simulink model "Braking_System_2021b"  (R2021b)
settings: Solver=VariableStepAuto  StartTime=0.0  StopTime=10.0  RelTol=1e-3
undefined symbols (not defined in the file): booster_calcData, booster_k1, booster_k2, Fp, frontBrake_cfrbr, lagtime, maitre_cyl_calcData, MR_trgtDecc_Unbrked, MR_trgtMass_Unbrked, Pa_max_ax, Pa_max_b, Pa_min_ax, Pa_min_b, pedale_calcData, pedale_Fr, pedale_method, pedale_Ratio_Test, pedale_Rp, pedale_TEST, Tf_ax, Tf_b, tracteur_chargeAR, tracteur_chargeAV, tracteur_h, tracteur_masseLaden, tracteur_masseLadenAR, tracteur_masseLadenAV, tracteur_masseUnladen, tracteur_masseUnladenAR, tracteur_masseUnladenAV, tracteur_maxRayAR, tracteur_maxRayAV, tracteur_minRayAR, tracteur_minRayAV, tracteur_RollRes, tracteur_x1, tracteur_x2, transmission_calcData, transmission_R4wd, transmission_Rbs, transmission_Redn_AV, transmission_Rend_AR, transmission_Rend_AV, transmission_Rfa, transmission_Rra, valve_hp_calcData, valve_hp_k1, valve_hp_k2, vitesse
libraries: simulink x2
settings Model: Creator=sb74808  LastModifiedBy=sb74808
settings DebuggingCC: UnconnectedInputMsg=none  UnconnectedOutputMsg=none  UnconnectedLineMsg=none
settings ModelReferenceCC: EnableRefExpFcnMdlSchedulingChecks=off
settings RTWCC: DLArmComputeVersion=20.02.1

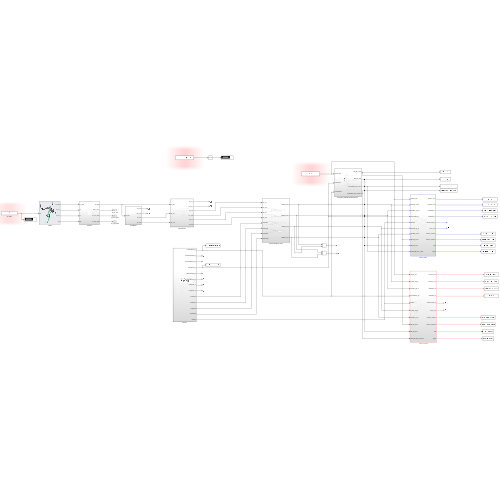
[thumbnail: Simulink's stored preview of the top-level diagram]
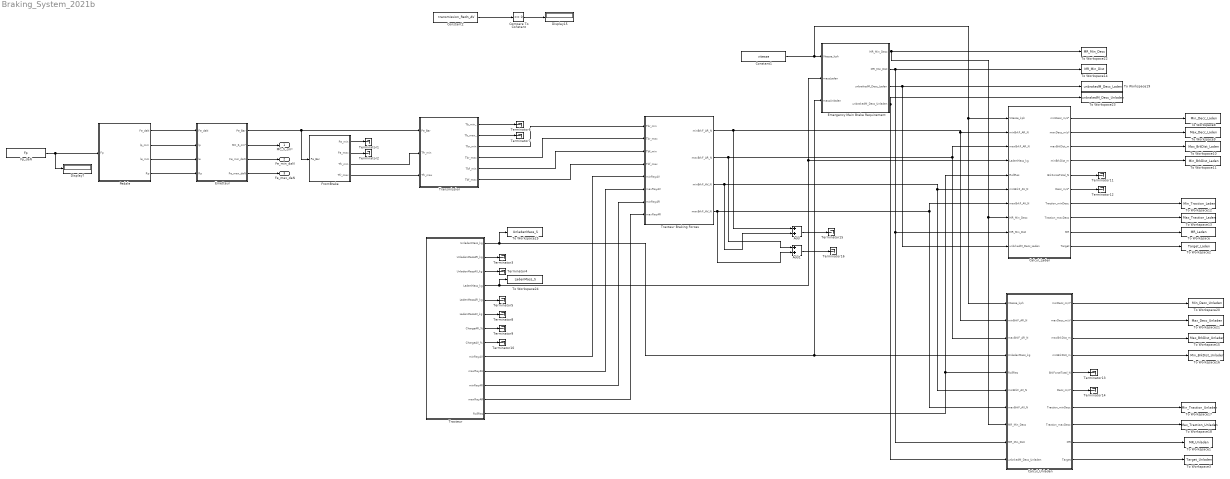
== system Braking_System_2021b ==
  Add : Sum
  Add1 : Sum
  Calcul_Laden : Subsystem
  Calcul_Unladen : Subsystem
  Compare To Constant : simulink/Logic and Bit Operations/Compare To Constant  relop===  const=0  OutDataTypeStr=boolean
  Constant1 : Constant  Value=vitesse
  Constant2 : Constant  Value=transmission_Redn_AV
  Display15 : Display
  Display7 : Display
  Emergency Main Brake Requirement : Subsystem
  Emetteur : Subsystem
  Fp_daN : Constant  Value=Fp
  FrontBrake : Subsystem
  Pedale : Subsystem
      mask Display: image('C:\Users\sb74808\OneDrive - AGCO Corp\Bureau\pedal.png'); % Use "Edit Image" on toolstrip to change.
  Terminator{1..16} (16 alike) : Terminator
  To Workspace : ToWorkspace  VariableName=MR_Laden  SaveFormat=Structure  SampleTime=-1
  To Workspace1 : ToWorkspace  VariableName=MR_Unladen  SaveFormat=Structure  SampleTime=-1
  To Workspace10 : ToWorkspace  VariableName=Max_BrkDist_Laden  SaveFormat=Structure  SampleTime=-1
  To Workspace11 : ToWorkspace  VariableName=Min_BrkDist_Laden  SaveFormat=Structure  SampleTime=-1
  To Workspace12 : ToWorkspace  VariableName=Min_Traction_Laden  SaveFormat=Structure  SampleTime=-1
      settings: Save2DSignal=2-D array (concatenate along first dimension)
  To Workspace13 : ToWorkspace  VariableName=Max_Traction_Laden  SaveFormat=Structure  SampleTime=-1
  To Workspace14 : ToWorkspace  VariableName=MR_Min_Dist  SaveFormat=Structure  SampleTime=-1
  To Workspace15 : ToWorkspace  VariableName=Max_BrkDist_Unladen  SaveFormat=Structure  SampleTime=-1
  To Workspace16 : ToWorkspace  VariableName=Min_BrkDist_Unladen  SaveFormat=Structure  SampleTime=-1
  To Workspace17 : ToWorkspace  VariableName=Min_Traction_Unladen  SaveFormat=Structure  SampleTime=-1
  To Workspace18 : ToWorkspace  VariableName=Max_Traction_Unladen  SaveFormat=Structure  SampleTime=-1
  To Workspace19 : ToWorkspace  VariableName=unbrakedM_Decc_Laden  SaveFormat=Structure  SampleTime=-1
  To Workspace2 : ToWorkspace  VariableName=Target_Laden  SaveFormat=Structure  SampleTime=-1
  To Workspace20 : ToWorkspace  VariableName=Min_Decc_Unladen  SaveFormat=Structure  SampleTime=-1
  To Workspace21 : ToWorkspace  VariableName=Max_Decc_Unladen  SaveFormat=Structure  SampleTime=-1
  To Workspace22 : ToWorkspace  VariableName=MR_Min_Decc  SaveFormat=Structure  SampleTime=-1
  To Workspace23 : ToWorkspace  VariableName=unbrakedM_Decc_Unladen  SaveFormat=Structure  SampleTime=-1
  To Workspace24 : ToWorkspace  VariableName=LadenMass_S  SaveFormat=Structure  SampleTime=-1
  To Workspace25 : ToWorkspace  VariableName=UnladenMass_S  SaveFormat=Structure  SampleTime=-1
  To Workspace3 : ToWorkspace  VariableName=Target_Unladen  SaveFormat=Structure  SampleTime=-1
  To Workspace8 : ToWorkspace  VariableName=Min_Decc_Laden  SaveFormat=Structure  SampleTime=-1
  To Workspace9 : ToWorkspace  VariableName=Max_Decc_Laden  SaveFormat=Structure  SampleTime=-1
  Tracteur : Subsystem
  Tracteur Braking Forces : Subsystem
  Transmission : Subsystem
  MC_S_cm² : Outport
  Fe_min_daN : Outport  Port=2
  Fe_max_daN : Outport  Port=3
  wires:
  Fp_daN/1 -> Pedale/1(Fp), Display7/1
  Pedale/2(lp_mm) -> Emetteur/2(lp)
  Pedale/3(le_mm) -> Emetteur/3(le)
  Pedale/4(Rp) -> Emetteur/4(Rp)
  Pedale/1(Fe_daN) -> Emetteur/1(Fe_daN)
  Emetteur/2(MC_S_cm²) -> MC_S_cm²/1
  Emetteur/3(Fe_min_daN) -> Fe_min_daN/1
  Emetteur/4(Fe_max_daN) -> Fe_max_daN/1
  Emetteur/1(Pe_Bar) -> FrontBrake/1(Pe_Bar), Transmission/1(Pe_Bar)
  FrontBrake/4(Tfr_max) -> Transmission/3(Tfr_max)
  FrontBrake/3(Tfr_min) -> Transmission/2(Tfr_min)
  Compare To Constant/1 -> Display15/1
  Constant2/1 -> Compare To Constant/1
  Transmission/3(Tbr_min) -> Tracteur Braking Forces/1(Tbr_min)
  Transmission/5(Tbf_min) -> Tracteur Braking Forces/3(Tbf_min)
  Transmission/6(Tbf_max) -> Tracteur Braking Forces/4(Tbf_max)
  Tracteur/9(minRayAV) -> Tracteur Braking Forces/5(minRayAV)
  Tracteur/10(maxRayAV) -> Tracteur Braking Forces/6(maxRayAV)
  Tracteur/11(minRayAR) -> Tracteur Braking Forces/7(minRayAR)
  Tracteur/12(maxRayAR) -> Tracteur Braking Forces/8(maxRayAR)
  Tracteur/13(RollRes) -> Calcul_Laden/5(RollRes), Calcul_Unladen/5(RollRes)
  Tracteur Braking Forces/1(minBrkF_AR_N) -> Add/1, Calcul_Unladen/2(minBrkF_AR_N), Calcul_Laden/2(minBrkF_AR_N)
  Tracteur Braking Forces/2(maxBrkF_AR_N) -> Calcul_Unladen/3(maxBrkF_AR_N), Calcul_Laden/3(maxBrkF_AR_N), Add1/1
  Tracteur Braking Forces/3(minBrkF_AV_N) -> Add/2, Calcul_Unladen/6(minBrkF_AV_N), Calcul_Laden/6(minBrkF_AV_N)
  Tracteur Braking Forces/4(maxBrkF_AV_N) -> Add1/2, Calcul_Unladen/7(maxBrkF_AV_N), Calcul_Laden/7(maxBrkF_AV_N)
  Transmission/1(Tb_min_) -> Terminator6/1
  Transmission/2(Tb_max_) -> Terminator7/1
  Transmission/4(Tbr_max) -> Tracteur Braking Forces/2(Tbr_max)
  Add/1 -> Terminator15/1
  Add1/1 -> Terminator16/1
  Constant1/1 -> Calcul_Unladen/1(Vitesse_kph), Calcul_Laden/1(Vitesse_kph), Emergency Main Brake Requirement/1(Vitesse_kph)
  Emergency Main Brake Requirement/1(MR_Min_Decc) -> To Workspace22/1, Calcul_Unladen/8(MR_Min_Decc), Calcul_Laden/8(MR_Min_Decc)
  Emergency Main Brake Requirement/2(MR_Min_Dist) -> To Workspace14/1, Calcul_Unladen/9(MR_Min_Dist), Calcul_Laden/9(MR_Min_Dist)
  Emergency Main Brake Requirement/3(unbrakedM_Decc_Laden) -> To Workspace19/1, Calcul_Laden/10(unbrkedM_Decc_Laden)
  Emergency Main Brake Requirement/4(unbrakedM_Decc_Unladen) -> To Workspace23/1, Calcul_Unladen/10(unbrkedM_Decc_Unladen)
  Calcul_Laden/1(minDecc_m/s²) -> To Workspace8/1
  Calcul_Laden/2(maxDecc_m/s²) -> To Workspace9/1
  Calcul_Laden/3(maxBrkDist_m) -> To Workspace10/1
  Calcul_Laden/4(minBrkDist_m) -> To Workspace11/1
  Calcul_Unladen/4(minBrkDist_m) -> To Workspace16/1
  Calcul_Unladen/3(maxBrkDist_m) -> To Workspace15/1
  Calcul_Unladen/2(maxDecc_m/s²) -> To Workspace21/1
  Calcul_Unladen/1(minDecc_m/s²) -> To Workspace20/1
  Tracteur/4(LadenMass_kg) -> Calcul_Laden/4(LadenMass_kg), Emergency Main Brake Requirement/2(massLaden), To Workspace24/1
  Tracteur/1(UnladenMass_kg) -> Calcul_Unladen/4(UnladenMass_kg), Emergency Main Brake Requirement/3(massUnladen), To Workspace25/1
  FrontBrake/1(Pa_min) -> Terminator1/1
  FrontBrake/2(Pa_max) -> Terminator2/1
  Tracteur/2(UnladenMassAR_kg) -> Terminator3/1
  Tracteur/3(UnladenMassAV_kg) -> Terminator4/1
  Tracteur/5(LadenMassAR_kg) -> Terminator5/1
  Tracteur/6(LadenMassAV_kg) -> Terminator8/1
  Tracteur/7(ChargeAR_%) -> Terminator9/1
  Tracteur/8(ChargeAV_%) -> Terminator10/1
  Calcul_Laden/5(BrkForceTotal_N) -> Terminator11/1
  Calcul_Laden/6(Decc_m/s²) -> Terminator12/1
  Calcul_Unladen/5(BrkForceTotal_N) -> Terminator13/1
  Calcul_Unladen/6(Decc_m/s²) -> Terminator14/1
  Calcul_Laden/9(MR) -> To Workspace/1
  Calcul_Laden/10(Target) -> To Workspace2/1
  Calcul_Laden/8(Traction_maxDecc) -> To Workspace13/1
  Calcul_Unladen/7(Traction_minDecc) -> To Workspace17/1
  Calcul_Unladen/8(Traction_maxDecc) -> To Workspace18/1
  Calcul_Unladen/9(MR) -> To Workspace1/1
  Calcul_Unladen/10(Target) -> To Workspace3/1
  Calcul_Laden/7(Traction_minDecc) -> To Workspace12/1

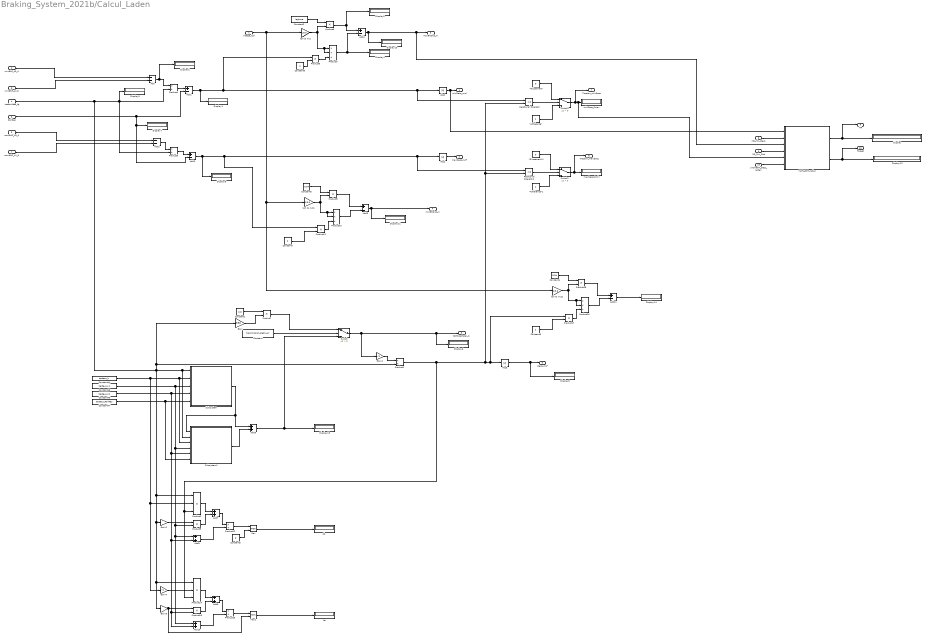
== system Braking_System_2021b/Calcul_Laden ==
  Vitesse_kph : Inport
  minBrkF_AR_N : Inport  Port=2
  maxBrkF_AR_N : Inport  Port=3
  LadenMass_kg : Inport  Port=4
  RollRes : Inport  Port=5
  minBrkF_AV_N : Inport  Port=6
  maxBrkF_AV_N : Inport  Port=7
  MR_Min_Decc : Inport  Port=8
  MR_Min_Dist : Inport  Port=9
  unbrkedM_Decc_Laden : Inport  Port=10
  "\"Adhérence\"" : Constant
  "\"Adhérence\"1" : Constant
  "\"Glissement\"" : Constant  Value=0
  "\"Glissement\"1" : Constant  Value=0
  Abs1 : Abs
  Abs2 : Abs
  Abs3 : Abs
  Add : Sum  Inputs=--
  Add{1,3..5,11} (5 alike) : Sum  Inputs=+-
  Add{6..10} (5 alike) : Sum
  Add2 : Sum  Inputs=--
  Constant : Constant  Value=transmission_Redn_AV
  Constant1 : Constant  Value=0.8
  Constant2 : Constant  Value=lagtime
  Constant3 : Constant  Value=0
  Constant4 : Constant  Value=0.54
  Constant44 : Constant  Value=tracteur_h
  Constant45 : Constant  Value=tracteur_x2
  Constant46 : Constant  Value=tracteur_x1
  Constant47 : Constant  Value=tracteur_RollRes
  Constant5 : Constant  Value=2
  Constant6 : Constant  Value=0.54
  Constant7 : Constant  Value=2
  Constant8 : Constant  Value=2
  Display{,1..14} (15 alike) : Display
  Gain : Gain  Gain=9.81
  Gain1 : Gain  Gain=-1
  Gain2 : Gain  Gain=9.81
  Gain3 : Gain  Gain=9.81
  Gain4 : Gain  Gain=-1
  MATLAB Function : MATLAB Function  TreatAsAtomicUnit=on
  Max : MinMax  Function=max  Inputs=2
  Max1 : MinMax  Inputs=2
  Na : Display
  Nb : Display
  Product{,3,6,8..9,11,15,17..18} (9 alike) : Product
  Product{1,4..5,12..13} (5 alike) : Product  Inputs=*/
  Product10 : Product  Inputs=**/
  Product14 : Product  Inputs=3
  Product16 : Product  Inputs=**/
  Product2 : Product  Inputs=3
  Product7 : Product  Inputs=**/
  Relational Operator : RelationalOperator  Operator=<=  OutDataTypeStr=boolean  RndMeth=Simplest
  Relational Operator1 : RelationalOperator  Operator=<=  OutDataTypeStr=boolean  RndMeth=Simplest
  Subsystem : Subsystem
  Subsystem1 : Subsystem
  Switch : Switch  Criteria=u2 > Threshold
  Switch1 : Switch  Criteria=u2 > Threshold
  Switch2 : Switch  Criteria=u2 > Threshold
  kph to m/s : Gain  Gain=1/3.6
  kph to m/s1 : Gain  Gain=1/3.6
  kph to m/s2 : Gain  Gain=1/3.6
  maxDecc_Pmin : Display
  minDecc_Pmax : Display
  minDecc_m/s² : Outport
  maxDecc_m/s² : Outport  Port=2
  maxBrkDist_m : Outport  Port=3
  minBrkDist_m : Outport  Port=4
  BrkForceTotal_N : Outport  Port=5
  Decc_m/s² : Outport  Port=6
  Traction_minDecc : Outport  Port=7
  Traction_maxDecc : Outport  Port=8
  MR : Outport  Port=9
  Target : Outport  Port=10
  wires:
  kph to m/s/1 -> Product7/1, Product7/2, Product6/2
  kph to m/s1/1 -> Product9/2, Product10/1, Product10/2
  Add/1 -> Display2/1, Product4/1
  Product9/1 -> Add5/1
  RollRes/1 -> Add3/2, Display7/1, Add1/2
  Product4/1 -> Add1/1
  Product6/1 -> Add4/1, Display5/1
  Constant5/1 -> Product8/2
  Constant2/1 -> Product6/1
  Product5/1 -> Add3/1
  Add4/1 -> MATLAB Function/3(maxBrkDist), maxBrkDist_m/1, Display10/1
  Add1/1 -> Relational Operator/1, Abs1/1, Product8/1, Display1/1
  Product8/1 -> Product7/3
  Add5/1 -> minBrkDist_m/1, Display11/1
  minBrkF_AV_N/1 -> Add/2
  Add2/1 -> Product5/1
  Constant7/1 -> Product11/2
  Product10/1 -> Add5/2
  Product11/1 -> Product10/3
  Constant6/1 -> Product9/1
  Product7/1 -> Add4/2, Display4/1
  maxBrkF_AR_N/1 -> Add2/1
  maxBrkF_AV_N/1 -> Add2/2
  minBrkF_AR_N/1 -> Add/1
  Subsystem/1(BrkRearForce) -> Subsystem1/1(BrkRearForce), Add6/1
  Constant47/1 -> Subsystem1/6(RollRes), Subsystem/5(RollRes)
  Subsystem1/1(BrkFrontForce) -> Add6/2
  Add6/1 -> Switch/3, Display13/1
  Gain/1 -> Product/2
  Constant1/1 -> Product/1
  Constant/1 -> Switch/2
  Product/1 -> Switch/1
  Switch/1 -> Display6/1, BrkForceTotal_N/1, Gain1/1
  Gain1/1 -> Product1/1
  Product2/1 -> Add7/1
  Product3/1 -> Add7/2
  Gain2/1 -> Product3/1
  Add7/1 -> Product12/1
  Add8/1 -> Product12/2
  Product12/1 -> Max/1
  Constant3/1 -> Max/2
  Max/1 -> Nb/1
  Add10/1 -> Product13/2
  Constant46/1 -> Subsystem1/4(X1), Add10/1, Add8/1, Product3/2, Subsystem/3(X1)
  Product14/1 -> Add9/1
  Product15/1 -> Add9/2
  Product13/1 -> Max1/1
  Add9/1 -> Product13/1
  Max1/1 -> Na/1
  Constant45/1 -> Product15/2, Add10/2, Add8/2, Subsystem1/5(X2), Subsystem/4(X2)
  Constant44/1 -> Gain4/1, Product2/2, Subsystem1/3(h), Subsystem/2(h)
  Gain3/1 -> Max1/2, Product15/1
  LadenMass_kg/1 -> Gain3/1, Product14/1, Gain2/1, Product2/1, Gain/1, Product1/2, Subsystem1/2(massLaden), Subsystem/1(massLaden), Product5/2, Product4/2, Display3/1
  Gain4/1 -> Product14/2
  Relational Operator/1 -> Switch1/2
  "\"Glissement\""/1 -> Switch1/1
  "\"Adhérence\""/1 -> Switch1/3
  Switch1/1 -> Traction_minDecc/1, MATLAB Function/5(Tract), minDecc_Pmax/1
  Switch2/1 -> Traction_maxDecc/1, maxDecc_Pmin/1
  "\"Adhérence\"1"/1 -> Switch2/3
  "\"Glissement\"1"/1 -> Switch2/1
  Relational Operator1/1 -> Switch2/2
  Product1/1 -> Relational Operator1/2, Relational Operator/2, Product17/1, Abs3/1, Product14/3, Product2/3
  Add3/1 -> Display9/1, Relational Operator1/1, Abs2/1, Product11/1
  MR_Min_Decc/1 -> MATLAB Function/2(MR_Min_Dec)
  MR_Min_Dist/1 -> MATLAB Function/4(MR_Min_Dist)
  unbrkedM_Decc_Laden/1 -> MATLAB Function/6(unbrk_M_Decc)
  MATLAB Function/1(MR) -> MR/1, Display/1
  MATLAB Function/2(Target) -> Target/1, Display12/1
  Abs1/1 -> MATLAB Function/1(minDecc), minDecc_m/s²/1
  Abs2/1 -> maxDecc_m/s²/1
  Abs3/1 -> Display8/1, Decc_m/s²/1
  Constant4/1 -> Product18/1
  Product17/1 -> Product16/3
  Product16/1 -> Add11/2
  Constant8/1 -> Product17/2
  Add11/1 -> Display14/1
  Vitesse_kph/1 -> kph to m/s2/1, kph to m/s1/1, kph to m/s/1
  Product18/1 -> Add11/1
  kph to m/s2/1 -> Product16/2, Product16/1, Product18/2

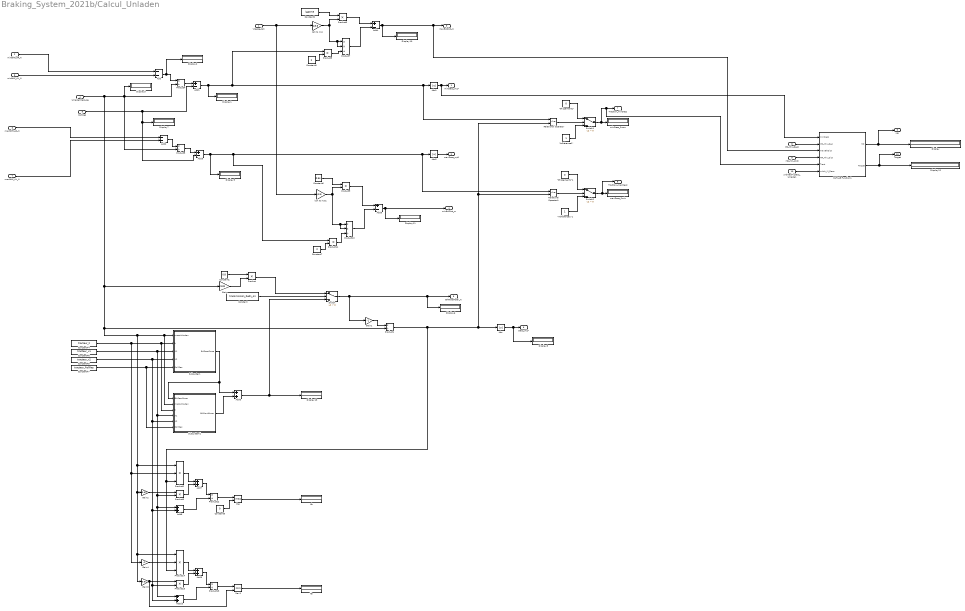
== system Braking_System_2021b/Calcul_Unladen ==
  Vitesse_kph : Inport
  minBrkF_AR_N : Inport  Port=2
  maxBrkF_AR_N : Inport  Port=3
  UnladenMass_kg : Inport  Port=4
  RollRes : Inport  Port=5
  minBrkF_AV_N : Inport  Port=6
  maxBrkF_AV_N : Inport  Port=7
  MR_Min_Decc : Inport  Port=8
  MR_Min_Dist : Inport  Port=9
  unbrkedM_Decc_Unladen : Inport  Port=10
  "\"Adhérence1\"" : Constant
  "\"Adhérence1\"1" : Constant
  "\"Glissement1\"" : Constant  Value=0
  "\"Glissement1\"1" : Constant  Value=0
  Abs : Abs
  Abs1 : Abs
  Abs2 : Abs
  Add : Sum  Inputs=--
  Add{1,3..5} (4 alike) : Sum  Inputs=+-
  Add{6..10} (5 alike) : Sum
  Add2 : Sum  Inputs=--
  Constant : Constant  Value=transmission_Redn_AV
  Constant1 : Constant  Value=0.8
  Constant2 : Constant  Value=lagtime
  Constant3 : Constant  Value=0
  Constant44 : Constant  Value=tracteur_h
  Constant45 : Constant  Value=tracteur_x2
  Constant46 : Constant  Value=tracteur_x1
  Constant47 : Constant  Value=tracteur_RollRes
  Constant5 : Constant  Value=2
  Constant6 : Constant  Value=0.54
  Constant7 : Constant  Value=2
  Display{,1..3,6..13} (12 alike) : Display
  Gain : Gain  Gain=9.81
  Gain1 : Gain  Gain=-1
  Gain2 : Gain  Gain=9.81
  Gain3 : Gain  Gain=9.81
  Gain4 : Gain  Gain=-1
  MATLAB Function1 : MATLAB Function  TreatAsAtomicUnit=on
  Max : MinMax  Function=max  Inputs=2
  Max1 : MinMax  Inputs=2
  Na : Display
  Nb : Display
  Product{,3,6,8..9,11,15} (7 alike) : Product
  Product{1,4..5,12..13} (5 alike) : Product  Inputs=*/
  Product10 : Product  Inputs=**/
  Product14 : Product  Inputs=3
  Product2 : Product  Inputs=3
  Product7 : Product  Inputs=**/
  Relational Operator : RelationalOperator  Operator=<=  OutDataTypeStr=boolean  RndMeth=Simplest
  Relational Operator1 : RelationalOperator  Operator=<=  OutDataTypeStr=boolean  RndMeth=Simplest
  Subsystem : Subsystem
  Subsystem1 : Subsystem
  Switch : Switch  Criteria=u2 > Threshold
  Switch1 : Switch  Criteria=u2 > Threshold
  Switch2 : Switch  Criteria=u2 > Threshold
  kph to m/s : Gain  Gain=1/3.6
  kph to m/s1 : Gain  Gain=1/3.6
  maxDecc_Pmin : Display
  minDecc_Pmax : Display
  minDecc_m/s² : Outport
  maxDecc_m/s² : Outport  Port=2
  maxBrkDist_m : Outport  Port=3
  minBrkDist_m : Outport  Port=4
  BrkForceTotal_N : Outport  Port=5
  Decc_m/s² : Outport  Port=6
  Traction_minDecc : Outport  Port=7
  Traction_maxDecc : Outport  Port=8
  MR : Outport  Port=9
  Target : Outport  Port=10
  wires:
  minBrkF_AR_N/1 -> Add/1
  maxBrkF_AV_N/1 -> Add2/2
  maxBrkF_AR_N/1 -> Add2/1
  Product7/1 -> Add4/2
  Constant6/1 -> Product9/1
  Product11/1 -> Product10/3
  Product10/1 -> Add5/2
  Constant7/1 -> Product11/2
  Add2/1 -> Product5/1
  minBrkF_AV_N/1 -> Add/2
  Add5/1 -> Display11/1, minBrkDist_m/1
  Product8/1 -> Product7/3
  Vitesse_kph/1 -> kph to m/s/1, kph to m/s1/1
  Product5/1 -> Add3/1
  Constant2/1 -> Product6/1
  Constant5/1 -> Product8/2
  Product6/1 -> Add4/1
  Product4/1 -> Add1/1
  RollRes/1 -> Display7/1, Add3/2, Add1/2
  Product9/1 -> Add5/1
  Add/1 -> Product4/1, Display2/1
  kph to m/s1/1 -> Product10/2, Product10/1, Product9/2
  kph to m/s/1 -> Product6/2, Product7/2, Product7/1
  Add3/1 -> Product11/1, Abs2/1, Relational Operator1/1, Display9/1
  "\"Glissement1\"1"/1 -> Switch2/1
  Relational Operator1/1 -> Switch2/2
  "\"Adhérence1\"1"/1 -> Switch2/3
  "\"Glissement1\""/1 -> Switch1/1
  Relational Operator/1 -> Switch1/2
  "\"Adhérence1\""/1 -> Switch1/3
  Product3/1 -> Add7/2
  Gain4/1 -> Product14/2
  Constant/1 -> Switch/2
  Product/1 -> Switch/1
  Gain3/1 -> Max1/2, Product15/1
  UnladenMass_kg/1 -> Product4/2, Display3/1, Product5/2, Gain/1, Product1/2, Gain3/1, Product14/1, Gain2/1, Product2/1, Subsystem1/2(massUnladen), Subsystem/1(massUnladen)
  Constant46/1 -> Subsystem1/4(X1), Add10/1, Add8/1, Product3/2, Subsystem/3(X1)
  Add8/1 -> Product12/2
  Constant1/1 -> Product/1
  Add7/1 -> Product12/1
  Product13/1 -> Max1/1
  Product14/1 -> Add9/1
  Max1/1 -> Na/1
  Gain2/1 -> Product3/1
  Subsystem1/1(BrkFrontForce) -> Add6/2
  Gain1/1 -> Product1/1
  Add10/1 -> Product13/2
  Add9/1 -> Product13/1
  Gain/1 -> Product/2
  Product15/1 -> Add9/2
  Product1/1 -> Relational Operator/2, Relational Operator1/2, Abs/1, Product14/3, Product2/3
  Switch/1 -> Display6/1, BrkForceTotal_N/1, Gain1/1
  Product2/1 -> Add7/1
  Constant45/1 -> Product15/2, Add10/2, Add8/2, Subsystem1/5(X2), Subsystem/4(X2)
  Product12/1 -> Max/1
  Add6/1 -> Switch/3, Display13/1
  Subsystem/1(BrkRearForce) -> Subsystem1/1(BrkRearForce), Add6/1
  Max/1 -> Nb/1
  Constant44/1 -> Gain4/1, Product2/2, Subsystem1/3(h), Subsystem/2(h)
  Constant3/1 -> Max/2
  Constant47/1 -> Subsystem1/6(RollRes), Subsystem/5(RollRes)
  Switch2/1 -> Traction_maxDecc/1, maxDecc_Pmin/1
  MR_Min_Decc/1 -> MATLAB Function1/2(MR_Min_Dec)
  unbrkedM_Decc_Unladen/1 -> MATLAB Function1/6(unbrk_M_Decc)
  MATLAB Function1/1(MR) -> MR/1, Display/1
  Switch1/1 -> MATLAB Function1/5(Tract), Traction_minDecc/1, minDecc_Pmax/1
  MATLAB Function1/2(Target) -> Target/1, Display12/1
  Add4/1 -> Display10/1, MATLAB Function1/3(maxBrkDist), maxBrkDist_m/1
  MR_Min_Dist/1 -> MATLAB Function1/4(MR_Min_Dist)
  Add1/1 -> Display1/1, Product8/1, Relational Operator/1, Abs1/1
  Abs1/1 -> MATLAB Function1/1(minDecc), minDecc_m/s²/1
  Abs2/1 -> maxDecc_m/s²/1
  Abs/1 -> Display8/1, Decc_m/s²/1

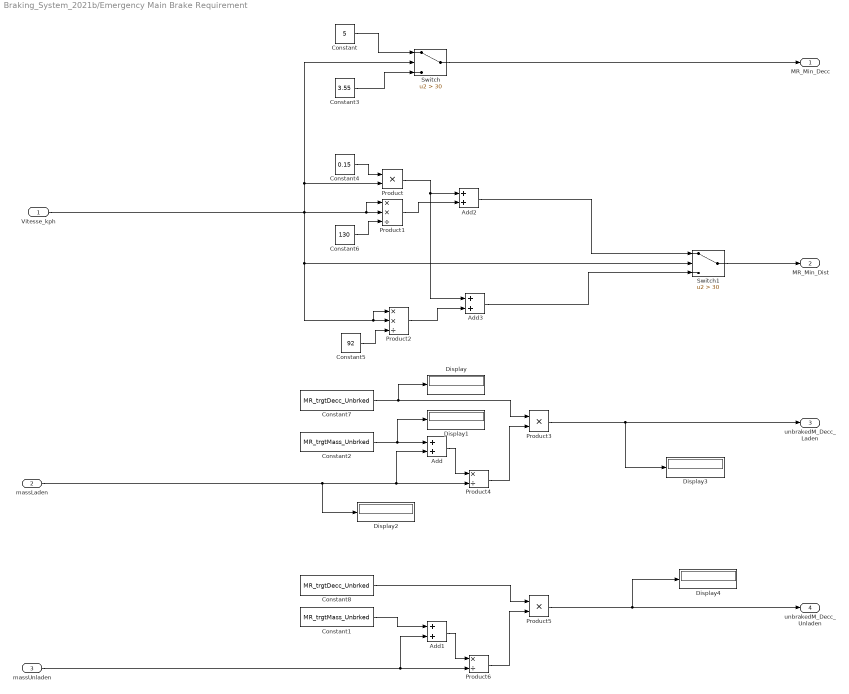
== system Braking_System_2021b/Emergency Main Brake Requirement ==
  Vitesse_kph : Inport
  massLaden : Inport  Port=2
  massUnladen : Inport  Port=3
  Add{,1..3} (4 alike) : Sum
  Constant : Constant  Value=5
  Constant1 : Constant  Value=MR_trgtMass_Unbrked
  Constant2 : Constant  Value=MR_trgtMass_Unbrked
  Constant3 : Constant  Value=3.55
  Constant4 : Constant  Value=0.15
  Constant5 : Constant  Value=92
  Constant6 : Constant  Value=130
  Constant7 : Constant  Value=MR_trgtDecc_Unbrked
  Constant8 : Constant  Value=MR_trgtDecc_Unbrked
  Display{,1..4} (5 alike) : Display
  Product : Product
  Product1 : Product  Inputs=**/
  Product2 : Product  Inputs=**/
  Product3 : Product  Inputs=**
  Product4 : Product  Inputs=*/
  Product5 : Product  Inputs=**
  Product6 : Product  Inputs=*/
  Switch : Switch  Criteria=u2 > Threshold  Threshold=30
  Switch1 : Switch  Criteria=u2 > Threshold  Threshold=30
  MR_Min_Decc : Outport
  MR_Min_Dist : Outport  Port=2
  unbrakedM_Decc_Laden : Outport  Port=3
  unbrakedM_Decc_Unladen : Outport  Port=4
  wires:
  Constant5/1 -> Product2/3
  Switch1/1 -> MR_Min_Dist/1
  Vitesse_kph/1 -> Product/2, Switch/2, Product2/2, Product2/1, Switch1/2, Product1/1, Product1/2
  Product/1 -> Add3/1, Add2/1
  Constant6/1 -> Product1/3
  Switch/1 -> MR_Min_Decc/1
  Product2/1 -> Add3/2
  Add3/1 -> Switch1/3
  Constant4/1 -> Product/1
  Add2/1 -> Switch1/1
  Product1/1 -> Add2/2
  Constant3/1 -> Switch/3
  Constant/1 -> Switch/1
  massLaden/1 -> Display2/1, Add/2, Product4/2
  Constant2/1 -> Display1/1, Add/1
  Product3/1 -> Display3/1, unbrakedM_Decc_Laden/1
  Add/1 -> Product4/1
  Product4/1 -> Product3/2
  Constant7/1 -> Display/1, Product3/1
  Constant8/1 -> Product5/1
  Product6/1 -> Product5/2
  Add1/1 -> Product6/1
  Product5/1 -> Display4/1, unbrakedM_Decc_Unladen/1
  Constant1/1 -> Add1/1
  massUnladen/1 -> Add1/2, Product6/2

== system Braking_System_2021b/Emetteur ==
  Fe_daN : Inport
  lp : Inport  Port=2
  le : Inport  Port=3
  Rp : Inport  Port=4
  Fe_max_daN_2 : Display
  Fe_min_daN_2 : Display
  MC_S_cm²_2 : Display
  Pe_Bar_2 : Display
  Terminator : Terminator
  Terminator1 : Terminator
  Terminator2 : Terminator
  Variant Subsystem : Subsystem  Variant=on
  Pe_Bar : Outport
  MC_S_cm² : Outport  Port=2
  Fe_min_daN : Outport  Port=3
  Fe_max_daN : Outport  Port=4
  wires:
  Fe_daN/1 -> Variant Subsystem/1(Fe_daN)
  lp/1 -> Terminator/1
  le/1 -> Terminator1/1
  Rp/1 -> Terminator2/1
  Variant Subsystem/2(MC_S_cm²) -> MC_S_cm²/1, MC_S_cm²_2/1
  Variant Subsystem/4(Fe_max_daN) -> Fe_max_daN/1, Fe_max_daN_2/1
  Variant Subsystem/3(Fe_min_daN) -> Fe_min_daN_2/1, Fe_min_daN/1
  Variant Subsystem/1(Pe_Bar) -> Pe_Bar/1, Pe_Bar_2/1

== system Braking_System_2021b/FrontBrake ==
  Pe_Bar : Inport
  Constant : Constant  Value=frontBrake_cfrbr
  Display : Display
  Eqn_Pa_max1 : Polyval  Coefs=[ Pa_max_ax, Pa_max_b ]
  Eqn_Pa_min1 : Polyval  Coefs=[Pa_min_ax, Pa_min_b ]
  Eqn_Tfr_max : Polyval  Coefs=[ Tf_ax, Tf_b ]
  Eqn_Tfr_min : Polyval  Coefs=[ Tf_ax, Tf_b ]
  Pa_max_1 : Display
  Pa_min_1 : Display
  Switch : Switch  Criteria=u2 > Threshold
  Tfr_max_2 : Display
  Tfr_min_3 : Display
  Pa_min : Outport
  Pa_max : Outport  Port=2
  Tfr_min : Outport  Port=3
  Tfr_max : Outport  Port=4
  wires:
  Eqn_Tfr_max/1 -> Tfr_max_2/1, Tfr_max/1
  Eqn_Pa_min1/1 -> Pa_min/1, Eqn_Tfr_min/1, Pa_min_1/1
  Eqn_Tfr_min/1 -> Tfr_min/1, Tfr_min_3/1
  Eqn_Pa_max1/1 -> Pa_max/1, Eqn_Tfr_max/1, Pa_max_1/1
  Constant/1 -> Display/1, Switch/3, Switch/2
  Pe_Bar/1 -> Switch/1
  Switch/1 -> Eqn_Pa_min1/1, Eqn_Pa_max1/1

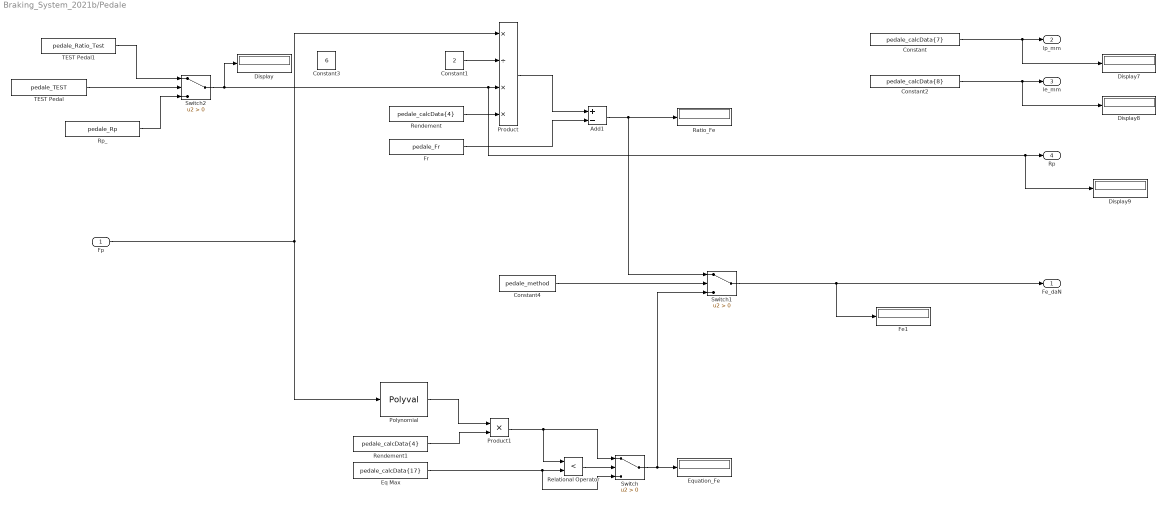
== system Braking_System_2021b/Pedale ==
  Fp : Inport
  Add1 : Sum  Inputs=+-
  Constant : Constant  Value=pedale_calcData{7}
  Constant1 : Constant  Value=2
  Constant2 : Constant  Value=pedale_calcData{8}
  Constant3 : Constant  Value=6
  Constant4 : Constant  Value=pedale_method
  Display{,7..9} (4 alike) : Display
  Eq Max : Constant  Value=pedale_calcData{17}
  Equation_Fe : Display
  Fe1 : Display
  Fr : Constant  Value=pedale_Fr
  Polynomial : Polyval  Coefs=[ pedale_calcData{13} pedale_calcData{14} pedale_calcData{15} ]
  Product : Product  Inputs=*/**
  Product1 : Product
  Ratio_Fe : Display
  Relational Operator : RelationalOperator  Operator=<  OutDataTypeStr=boolean  RndMeth=Simplest
  Rendement : Constant  Value=pedale_calcData{4}
  Rendement1 : Constant  Value=pedale_calcData{4}
  Rp_ : Constant  Value=pedale_Rp
  Switch : Switch  Criteria=u2 > Threshold
  Switch1 : Switch  Criteria=u2 > Threshold
  Switch2 : Switch  Criteria=u2 > Threshold
  TEST Pedal : Constant  Value=pedale_TEST
  TEST Pedal1 : Constant  Value=pedale_Ratio_Test
  Fe_daN : Outport
  lp_mm : Outport  Port=2
  le_mm : Outport  Port=3
  Rp : Outport  Port=4
  wires:
  Constant2/1 -> le_mm/1, Display8/1
  Constant1/1 -> Product/2
  Add1/1 -> Switch1/1, Ratio_Fe/1
  Eq Max/1 -> Switch/3, Relational Operator/2
  Constant/1 -> lp_mm/1, Display7/1
  Product/1 -> Add1/1
  Switch/1 -> Switch1/3, Equation_Fe/1
  Relational Operator/1 -> Switch/2
  Fr/1 -> Add1/2
  Polynomial/1 -> Product1/1
  Fp/1 -> Product/1, Polynomial/1
  Switch1/1 -> Fe_daN/1, Fe1/1
  Rendement1/1 -> Product1/2
  Rendement/1 -> Product/4
  Product1/1 -> Switch/1, Relational Operator/1
  Switch2/1 -> Display/1, Display9/1, Rp/1, Product/3
  Constant4/1 -> Switch1/2
  TEST Pedal/1 -> Switch2/2
  Rp_/1 -> Switch2/3
  TEST Pedal1/1 -> Switch2/1

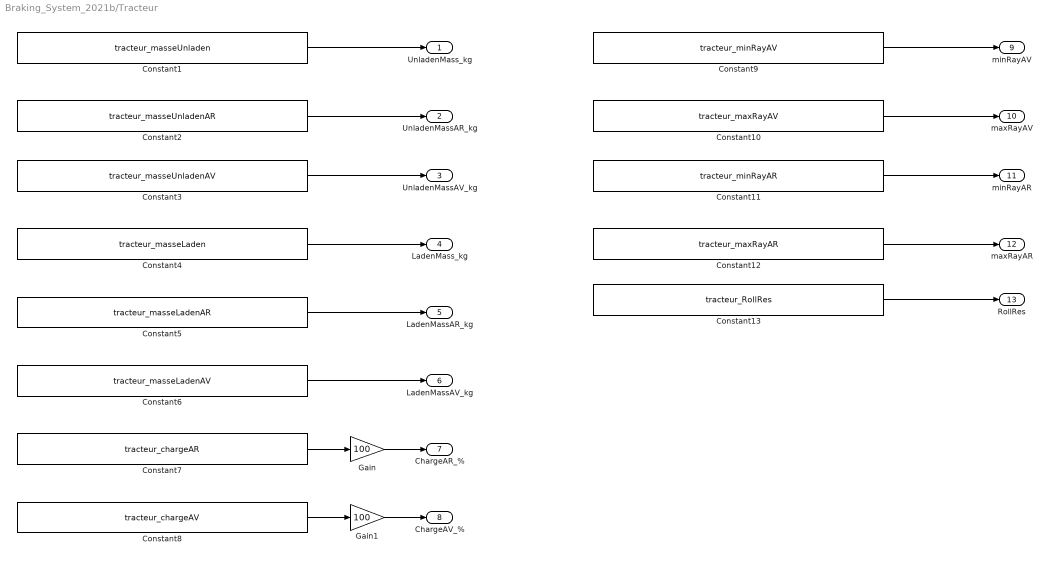
== system Braking_System_2021b/Tracteur ==
  Constant1 : Constant  Value=tracteur_masseUnladen
  Constant10 : Constant  Value=tracteur_maxRayAV
  Constant11 : Constant  Value=tracteur_minRayAR
  Constant12 : Constant  Value=tracteur_maxRayAR
  Constant13 : Constant  Value=tracteur_RollRes
  Constant2 : Constant  Value=tracteur_masseUnladenAR
  Constant3 : Constant  Value=tracteur_masseUnladenAV
  Constant4 : Constant  Value=tracteur_masseLaden
  Constant5 : Constant  Value=tracteur_masseLadenAR
  Constant6 : Constant  Value=tracteur_masseLadenAV
  Constant7 : Constant  Value=tracteur_chargeAR
  Constant8 : Constant  Value=tracteur_chargeAV
  Constant9 : Constant  Value=tracteur_minRayAV
  Gain : Gain  Gain=100
  Gain1 : Gain  Gain=100
  UnladenMass_kg : Outport
  UnladenMassAR_kg : Outport  Port=2
  UnladenMassAV_kg : Outport  Port=3
  LadenMass_kg : Outport  Port=4
  LadenMassAR_kg : Outport  Port=5
  LadenMassAV_kg : Outport  Port=6
  ChargeAR_% : Outport  Port=7
  ChargeAV_% : Outport  Port=8
  minRayAV : Outport  Port=9
  maxRayAV : Outport  Port=10
  minRayAR : Outport  Port=11
  maxRayAR : Outport  Port=12
  RollRes : Outport  Port=13
  wires:
  Constant2/1 -> UnladenMassAR_kg/1
  Constant3/1 -> UnladenMassAV_kg/1
  Constant4/1 -> LadenMass_kg/1
  Constant5/1 -> LadenMassAR_kg/1
  Constant6/1 -> LadenMassAV_kg/1
  Constant7/1 -> Gain/1
  Constant8/1 -> Gain1/1
  Constant1/1 -> UnladenMass_kg/1
  Gain/1 -> ChargeAR_%/1
  Gain1/1 -> ChargeAV_%/1
  Constant9/1 -> minRayAV/1
  Constant10/1 -> maxRayAV/1
  Constant11/1 -> minRayAR/1
  Constant12/1 -> maxRayAR/1
  Constant13/1 -> RollRes/1

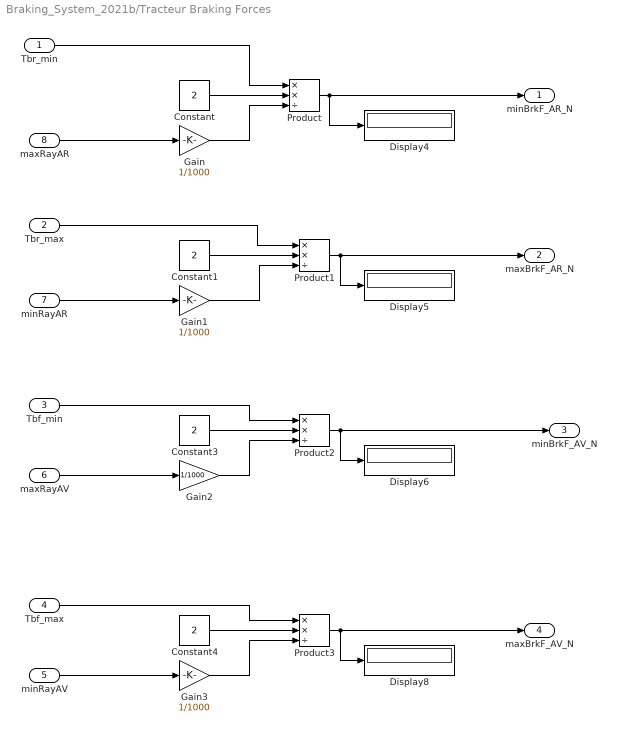
== system Braking_System_2021b/Tracteur Braking Forces ==
  Tbr_min : Inport
  Tbr_max : Inport  Port=2
  Tbf_min : Inport  Port=3
  Tbf_max : Inport  Port=4
  minRayAV : Inport  Port=5
  maxRayAV : Inport  Port=6
  minRayAR : Inport  Port=7
  maxRayAR : Inport  Port=8
  Constant{,1,3..4} (4 alike) : Constant  Value=2
  Display{4..6,8} (4 alike) : Display
  Gain{,1..3} (4 alike) : Gain  Gain=1/1000
  Product{,1..3} (4 alike) : Product  Inputs=**/
  minBrkF_AR_N : Outport
  maxBrkF_AR_N : Outport  Port=2
  minBrkF_AV_N : Outport  Port=3
  maxBrkF_AV_N : Outport  Port=4
  wires:
  Constant1/1 -> Product1/2
  Product2/1 -> minBrkF_AV_N/1, Display6/1
  Product/1 -> minBrkF_AR_N/1, Display4/1
  Constant/1 -> Product/2
  Gain2/1 -> Product2/3
  Tbr_max/1 -> Product1/1
  Product3/1 -> maxBrkF_AV_N/1, Display8/1
  Gain1/1 -> Product1/3
  Tbf_min/1 -> Product2/1
  Constant3/1 -> Product2/2
  Product1/1 -> maxBrkF_AR_N/1, Display5/1
  Gain/1 -> Product/3
  Constant4/1 -> Product3/2
  Gain3/1 -> Product3/3
  minRayAV/1 -> Gain3/1
  maxRayAV/1 -> Gain2/1
  Tbr_min/1 -> Product/1
  minRayAR/1 -> Gain1/1
  maxRayAR/1 -> Gain/1
  Tbf_max/1 -> Product3/1

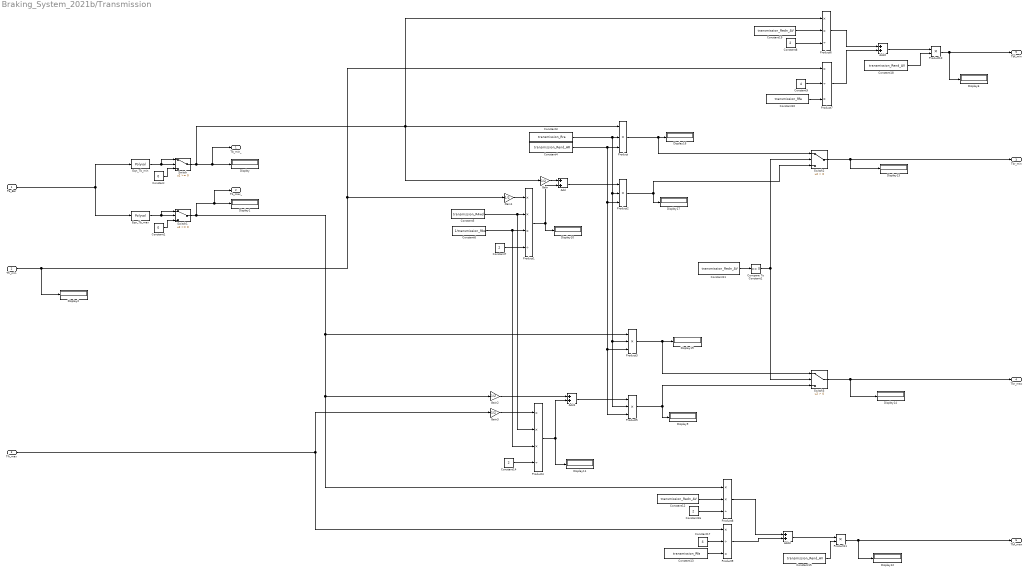
== system Braking_System_2021b/Transmission ==
  Pe_Bar : Inport
  Tfr_min : Inport  Port=2
  Tfr_max : Inport  Port=3
  Add{,1..3} (4 alike) : Sum
  Compare To Constant1 : simulink/Logic and Bit Operations/Compare To Constant  relop===  const=0  OutDataTypeStr=boolean
  Constant : Constant  Value=0
  Constant1 : Constant  Value=0
  Constant10 : Constant  Value=transmission_Rfa
  Constant11 : Constant  Value=transmission_Redn_AV
  Constant12 : Constant  Value=transmission_Redn_AV
  Constant13 : Constant  Value=transmission_Rfa
  Constant{7..8,14,16} (4 alike) : Constant  Value=2
  Constant15 : Constant  Value=transmission_Rend_AV
  Constant17 : Constant  Value=4
  Constant18 : Constant  Value=transmission_Rend_AV
  Constant19 : Constant  Value=transmission_Redn_AV
  Constant3 : Constant  Value=transmission_Rra
  Constant4 : Constant  Value=transmission_Rend_AR
  Constant5 : Constant  Value=transmission_R4wd
  Constant6 : Constant  Value=1/transmission_Rbs
  Constant9 : Constant  Value=4
  Display{,1..2,6,9..14,16..17,19} (13 alike) : Display
  Eqn_Tb_max : Polyval  Coefs=[ transmission_calcData{14}, transmission_calcData{15}, transmission_calcData{16}, transmission_calcData{17} ]
  Eqn_Tb_min : Polyval  Coefs=[ transmission_calcData{10}, transmission_calcData{11}, transmission_calcData{12}, transmission_calcData{13}]
  Gain{,1..3} (4 alike) : Gain  Gain=1/2
  Product{,2..3,5} (4 alike) : Product  Inputs=3
  Product1 : Product  Inputs=***/
  Product10 : Product
  Product11 : Product
  Product4 : Product  Inputs=***/
  Product6 : Product  Inputs=**/
  Product7 : Product  Inputs=*/*
  Product8 : Product  Inputs=**/
  Product9 : Product  Inputs=*/*
  Switch : Switch
  Switch1 : Switch
  Switch2 : Switch  Criteria=u2 > Threshold
  Switch3 : Switch  Criteria=u2 > Threshold
  Tb_min_ : Outport
  Tb_max_ : Outport  Port=2
  Tbr_min : Outport  Port=3
  Tbr_max : Outport  Port=4
  Tbf_min : Outport  Port=5
  Tbf_max : Outport  Port=6
  wires:
  Constant11/1 -> Compare To Constant1/1
  Switch/1 -> Display/1, Tb_min_/1, Product6/1, Gain/1, Product/1
  Constant3/1 -> Product5/2, Product3/2, Product2/2, Product/2
  Eqn_Tb_max/1 -> Switch1/2, Switch1/1
  Constant6/1 -> Product4/3, Product1/3
  Pe_Bar/1 -> Eqn_Tb_min/1, Eqn_Tb_max/1
  Product11/1 -> Tbf_max/1, Display12/1
  Eqn_Tb_min/1 -> Switch/1, Switch/2
  Constant1/1 -> Switch1/3
  Product2/1 -> Display17/1, Switch2/3
  Tfr_max/1 -> Product9/1, Gain3/1
  Product5/1 -> Switch3/3, Display9/1
  Product3/1 -> Switch3/1, Display19/1
  Gain2/1 -> Add1/1
  Constant18/1 -> Product10/2
  Switch2/1 -> Tbr_min/1, Display13/1
  Compare To Constant1/1 -> Switch2/2, Switch3/2
  Add/1 -> Product2/1
  Constant13/1 -> Product9/3
  Add3/1 -> Product11/1
  Constant8/1 -> Product6/3
  Constant/1 -> Switch/3
  Constant14/1 -> Product4/4
  Switch1/1 -> Gain2/1, Product8/1, Product3/1, Tb_max_/1, Display1/1
  Product10/1 -> Display6/1, Tbf_min/1
  Constant12/1 -> Product8/2
  Constant16/1 -> Product8/3
  Constant4/1 -> Product5/3, Product3/3, Product2/3, Product/3
  Constant17/1 -> Product9/2
  Product8/1 -> Add3/1
  Product9/1 -> Add3/2
  Constant5/1 -> Product4/2, Product1/2
  Product7/1 -> Add2/2
  Product4/1 -> Add1/2, Display11/1
  Switch3/1 -> Tbr_max/1, Display14/1
  Add2/1 -> Product10/1
  Product6/1 -> Add2/1
  Add1/1 -> Product5/1
  Gain1/1 -> Product1/1
  Constant7/1 -> Product1/4
  Constant19/1 -> Product6/2
  Tfr_min/1 -> Display2/1, Product7/1, Gain1/1
  Constant9/1 -> Product7/2
  Constant10/1 -> Product7/3
  Gain/1 -> Add/1
  Product/1 -> Switch2/1, Display16/1
  Gain3/1 -> Product4/1
  Product1/1 -> Display10/1, Add/2
  Constant15/1 -> Product11/2

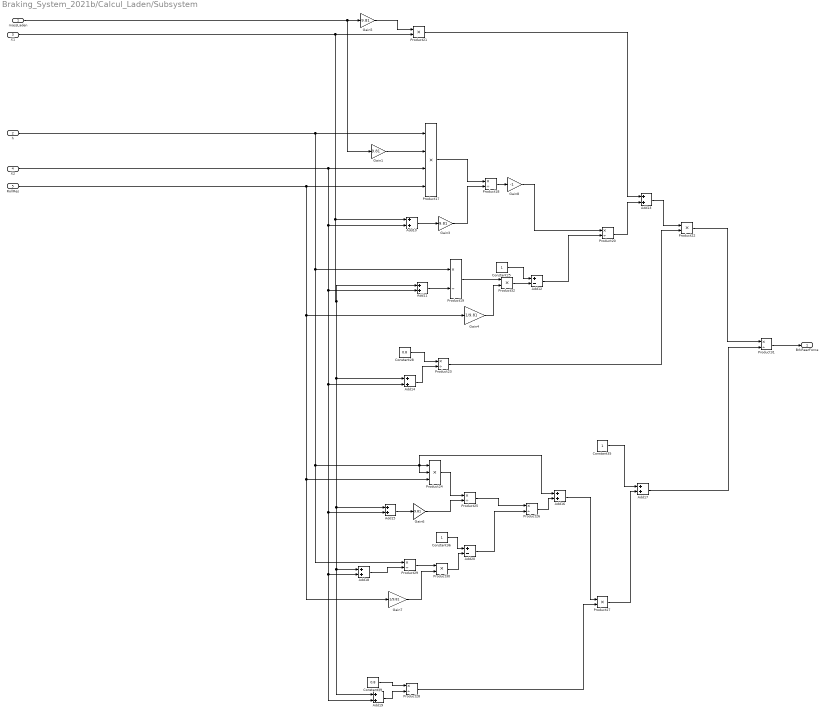
== system Braking_System_2021b/Calcul_Laden/Subsystem ==
  massLaden : Inport
  h : Inport  Port=2
  X1 : Inport  Port=3
  X2 : Inport  Port=4
  RollRes : Inport  Port=5
  Add{10..11,13..19} (9 alike) : Sum
  Add12 : Sum  Inputs=+-
  Add20 : Sum  Inputs=+-
  Constant25 : Constant
  Constant28 : Constant  Value=0.8
  Constant35 : Constant
  Constant36 : Constant
  Constant39 : Constant  Value=0.8
  Gain{1,3,5..6} (4 alike) : Gain  Gain=9.81
  Gain4 : Gain  Gain=1/9.81
  Gain7 : Gain  Gain=1/9.81
  Gain8 : Gain  Gain=-1
  Product17 : Product  Inputs=4
  Product{18..20,23,25..26,28..29,31} (9 alike) : Product  Inputs=*/
  Product{21..22,27,32} (4 alike) : Product
  Product24 : Product  Inputs=3
  Product30 : Product  Inputs=**
  BrkRearForce : Outport
  wires:
  Constant28/1 -> Product23/1
  Gain8/1 -> Product20/1
  massLaden/1 -> Gain1/1, Gain5/1
  Add11/1 -> Product19/2
  Product30/1 -> Add20/2
  Add18/1 -> Product29/2
  Constant39/1 -> Product28/1
  Add19/1 -> Product28/2
  Product32/1 -> Add12/2
  Product25/1 -> Product26/1
  Constant36/1 -> Add20/1
  Product19/1 -> Product32/1
  Constant25/1 -> Add12/1
  Product23/1 -> Product22/2
  Add16/1 -> Product27/1
  Add20/1 -> Product26/2
  Gain4/1 -> Product32/2
  Product28/1 -> Product27/2
  Add12/1 -> Product20/2
  Product27/1 -> Add17/2
  Gain7/1 -> Product30/2
  Product22/1 -> Product31/1
  Gain1/1 -> Product17/2
  Product21/1 -> Add13/1
  Add13/1 -> Product22/1
  Add14/1 -> Product23/2
  Product18/1 -> Gain8/1
  RollRes/1 -> Gain7/1, Product24/3, Gain4/1, Product17/4
  X2/1 -> Add19/2, Add18/2, Add15/2, Add14/2, Add11/2, Add10/2, Product17/3
  Product20/1 -> Add13/2
  X1/1 -> Add14/1, Add18/1, Add19/1, Add15/1, Add11/1, Add10/1, Product21/2
  Gain3/1 -> Product18/2
  Product24/1 -> Product25/1
  Add15/1 -> Gain6/1
  Add10/1 -> Gain3/1
  Gain6/1 -> Product25/2
  Add17/1 -> Product31/2
  Product29/1 -> Product30/1
  Gain5/1 -> Product21/1
  h/1 -> Add16/1, Product24/2, Product24/1, Product29/1, Product19/1, Product17/1
  Constant35/1 -> Add17/1
  Product26/1 -> Add16/2
  Product17/1 -> Product18/1
  Product31/1 -> BrkRearForce/1

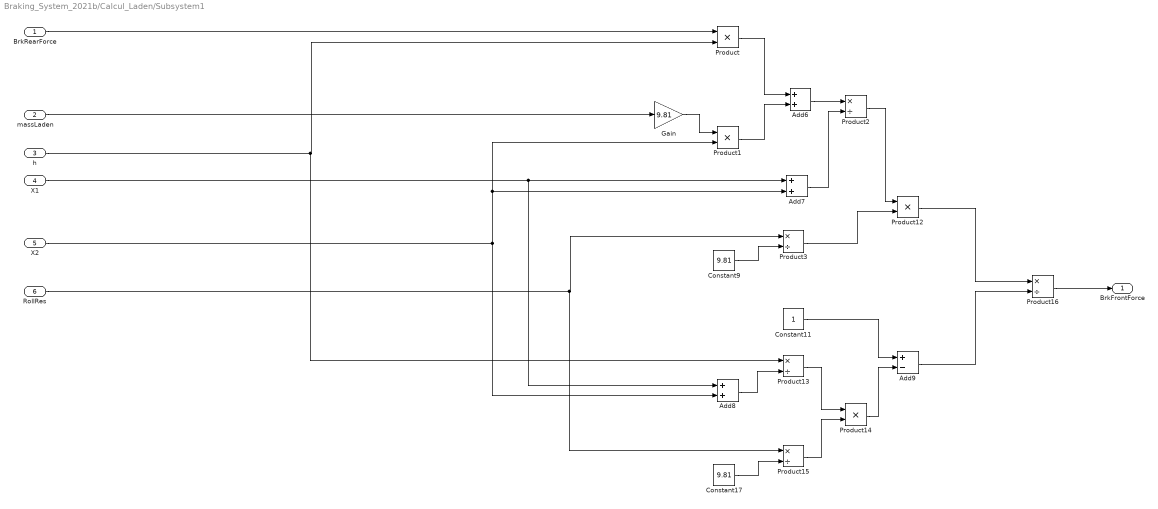
== system Braking_System_2021b/Calcul_Laden/Subsystem1 ==
  BrkRearForce : Inport
  massLaden : Inport  Port=2
  h : Inport  Port=3
  X1 : Inport  Port=4
  X2 : Inport  Port=5
  RollRes : Inport  Port=6
  Add6 : Sum
  Add7 : Sum
  Add8 : Sum
  Add9 : Sum  Inputs=+-
  Constant11 : Constant
  Constant17 : Constant  Value=9.81
  Constant9 : Constant  Value=9.81
  Gain : Gain  Gain=9.81
  Product : Product
  Product1 : Product
  Product12 : Product
  Product{2..3,13,15..16} (5 alike) : Product  Inputs=*/
  Product14 : Product  Inputs=**
  BrkFrontForce : Outport
  wires:
  Product3/1 -> Product12/2
  Product15/1 -> Product14/2
  Product2/1 -> Product12/1
  Add8/1 -> Product13/2
  Product14/1 -> Add9/2
  Add9/1 -> Product16/2
  Product/1 -> Add6/1
  Product16/1 -> BrkFrontForce/1
  Gain/1 -> Product1/1
  Constant9/1 -> Product3/2
  Product12/1 -> Product16/1
  Add7/1 -> Product2/2
  RollRes/1 -> Product15/1, Product3/1
  massLaden/1 -> Gain/1
  h/1 -> Product13/1, Product/2
  Add6/1 -> Product2/1
  Constant11/1 -> Add9/1
  Product1/1 -> Add6/2
  Constant17/1 -> Product15/2
  Product13/1 -> Product14/1
  X1/1 -> Add8/1, Add7/1
  X2/1 -> Add8/2, Add7/2, Product1/2
  BrkRearForce/1 -> Product/1

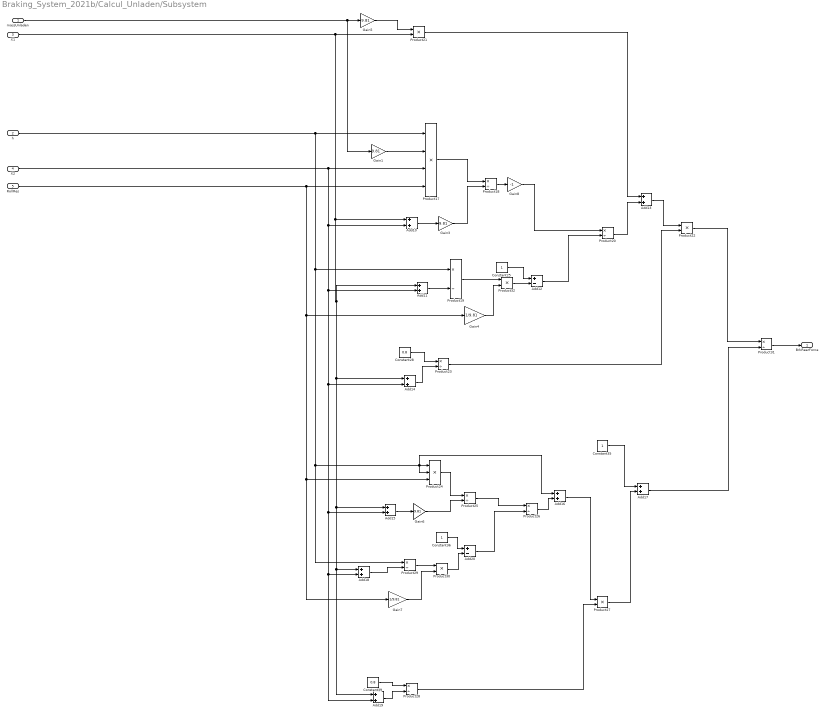
== system Braking_System_2021b/Calcul_Unladen/Subsystem ==
  massUnladen : Inport
  h : Inport  Port=2
  X1 : Inport  Port=3
  X2 : Inport  Port=4
  RollRes : Inport  Port=5
  Add{10..11,13..19} (9 alike) : Sum
  Add12 : Sum  Inputs=+-
  Add20 : Sum  Inputs=+-
  Constant25 : Constant
  Constant28 : Constant  Value=0.8
  Constant35 : Constant
  Constant36 : Constant
  Constant39 : Constant  Value=0.8
  Gain{1,3,5..6} (4 alike) : Gain  Gain=9.81
  Gain4 : Gain  Gain=1/9.81
  Gain7 : Gain  Gain=1/9.81
  Gain8 : Gain  Gain=-1
  Product17 : Product  Inputs=4
  Product{18..20,23,25..26,28..29,31} (9 alike) : Product  Inputs=*/
  Product{21..22,27,32} (4 alike) : Product
  Product24 : Product  Inputs=3
  Product30 : Product  Inputs=**
  BrkRearForce : Outport
  wires:
  Constant28/1 -> Product23/1
  Gain8/1 -> Product20/1
  massUnladen/1 -> Gain1/1, Gain5/1
  Add11/1 -> Product19/2
  Product30/1 -> Add20/2
  Add18/1 -> Product29/2
  Constant39/1 -> Product28/1
  Add19/1 -> Product28/2
  Product32/1 -> Add12/2
  Product25/1 -> Product26/1
  Constant36/1 -> Add20/1
  Product19/1 -> Product32/1
  Constant25/1 -> Add12/1
  Product23/1 -> Product22/2
  Add16/1 -> Product27/1
  Add20/1 -> Product26/2
  Gain4/1 -> Product32/2
  Product28/1 -> Product27/2
  Add12/1 -> Product20/2
  Product27/1 -> Add17/2
  Gain7/1 -> Product30/2
  Product22/1 -> Product31/1
  Gain1/1 -> Product17/2
  Product21/1 -> Add13/1
  Add13/1 -> Product22/1
  Add14/1 -> Product23/2
  Product18/1 -> Gain8/1
  RollRes/1 -> Gain7/1, Product24/3, Gain4/1, Product17/4
  X2/1 -> Add19/2, Add18/2, Add15/2, Add14/2, Add11/2, Add10/2, Product17/3
  Product20/1 -> Add13/2
  X1/1 -> Add14/1, Add18/1, Add19/1, Add15/1, Add11/1, Add10/1, Product21/2
  Gain3/1 -> Product18/2
  Product24/1 -> Product25/1
  Add15/1 -> Gain6/1
  Add10/1 -> Gain3/1
  Gain6/1 -> Product25/2
  Add17/1 -> Product31/2
  Product29/1 -> Product30/1
  Gain5/1 -> Product21/1
  h/1 -> Add16/1, Product24/2, Product24/1, Product29/1, Product19/1, Product17/1
  Constant35/1 -> Add17/1
  Product26/1 -> Add16/2
  Product17/1 -> Product18/1
  Product31/1 -> BrkRearForce/1

== system Braking_System_2021b/Calcul_Unladen/Subsystem1 ==
  BrkRearForce : Inport
  massUnladen : Inport  Port=2
  h : Inport  Port=3
  X1 : Inport  Port=4
  X2 : Inport  Port=5
  RollRes : Inport  Port=6
  Add6 : Sum
  Add7 : Sum
  Add8 : Sum
  Add9 : Sum  Inputs=+-
  Constant11 : Constant
  Constant17 : Constant  Value=9.81
  Constant9 : Constant  Value=9.81
  Gain : Gain  Gain=9.81
  Product : Product
  Product1 : Product
  Product12 : Product
  Product{2..3,13,15..16} (5 alike) : Product  Inputs=*/
  Product14 : Product  Inputs=**
  BrkFrontForce : Outport
  wires:
  Product3/1 -> Product12/2
  Product15/1 -> Product14/2
  Product2/1 -> Product12/1
  Add8/1 -> Product13/2
  Product14/1 -> Add9/2
  Add9/1 -> Product16/2
  Product/1 -> Add6/1
  Product16/1 -> BrkFrontForce/1
  Gain/1 -> Product1/1
  Constant9/1 -> Product3/2
  Product12/1 -> Product16/1
  Add7/1 -> Product2/2
  RollRes/1 -> Product15/1, Product3/1
  massUnladen/1 -> Gain/1
  h/1 -> Product13/1, Product/2
  Add6/1 -> Product2/1
  Constant11/1 -> Add9/1
  Product1/1 -> Add6/2
  Constant17/1 -> Product15/2
  Product13/1 -> Product14/1
  X1/1 -> Add8/1, Add7/1
  X2/1 -> Add8/2, Add7/2, Product1/2
  BrkRearForce/1 -> Product/1

== system Braking_System_2021b/Emetteur/Variant Subsystem ==
  note: 1) Add Subsystem or Model blocks as valid variant choices.
      | 2) You cannot connect blocks at this level. At simulation, connectivity is automatically
      | determined, based on the active variant and port name matching.
  Fe_daN : Inport
  Booster : Subsystem  VariantControl=emetteur_Sel == 2
  Maitre_Cylindre : Subsystem  VariantControl=emetteur_Sel == 1
  Valve_HP : Subsystem  VariantControl=emetteur_Sel == 3
  Pe_Bar : Outport
  MC_S_cm² : Outport  Port=2
  Fe_min_daN : Outport  Port=3
  Fe_max_daN : Outport  Port=4

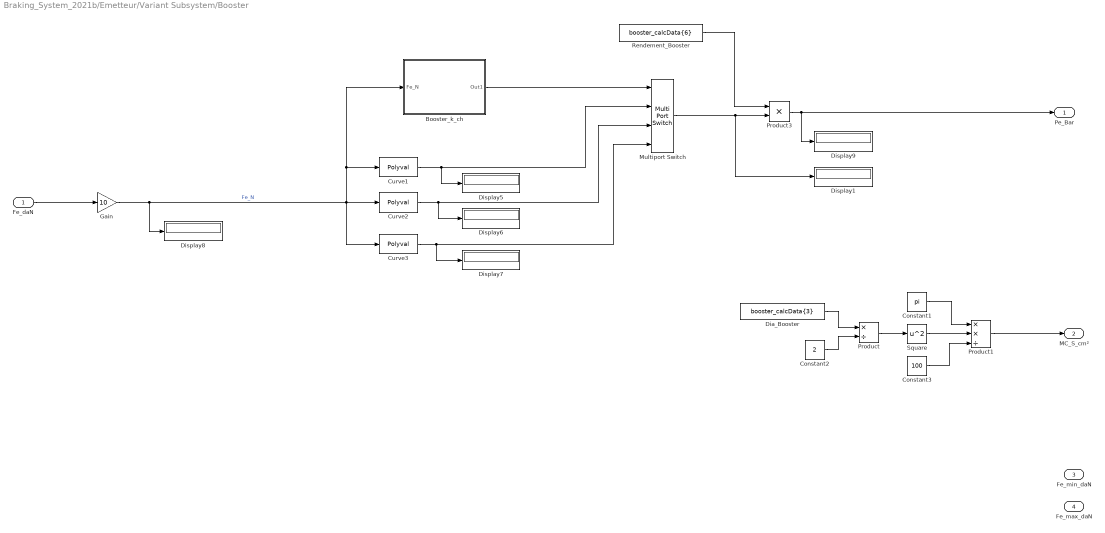
== system Braking_System_2021b/Emetteur/Variant Subsystem/Booster ==
  Fe_daN : Inport
  Booster_k_ch : Subsystem
  Constant1 : Constant  Value=pi
  Constant2 : Constant  Value=2
  Constant3 : Constant  Value=100
  Curve1 : Polyval  Coefs=[booster_calcData{7}, booster_calcData{8}, booster_calcData{9} ]
  Curve2 : Polyval  Coefs=[booster_calcData{10}, booster_calcData{11}, booster_calcData{12} ]
  Curve3 : Polyval  Coefs=[booster_calcData{14}, booster_calcData{15}, booster_calcData{16} ]
  Dia_Booster : Constant  Value=booster_calcData{3}
  Display{1,5..9} (6 alike) : Display
  Gain : Gain  Gain=10
  Multiport Switch : MultiPortSwitch
  Product : Product  Inputs=*/
  Product1 : Product  Inputs=**/
  Product3 : Product
  Rendement_Booster : Constant  Value=booster_calcData{6}
  Square : Math  Operator=square  SaturateOnIntegerOverflow=on
  Pe_Bar : Outport
  MC_S_cm² : Outport  Port=2
  Fe_min_daN : Outport  Port=3
  Fe_max_daN : Outport  Port=4
  wires:
  Booster_k_ch/1(Out1) -> Multiport Switch/1
  Square/1 -> Product1/2
  Constant2/1 -> Product/2
  Constant1/1 -> Product1/1
  Curve2/1 -> Display6/1, Multiport Switch/3
  Dia_Booster/1 -> Product/1
  Curve1/1 -> Display5/1, Multiport Switch/2
  Gain/1 -> Curve3/1, Booster_k_ch/1(Fe_N), Curve1/1, Curve2/1, Display8/1  "Fe_N"
  Product1/1 -> MC_S_cm²/1
  Constant3/1 -> Product1/3
  Rendement_Booster/1 -> Product3/1
  Product/1 -> Square/1
  Fe_daN/1 -> Gain/1
  Product3/1 -> Pe_Bar/1, Display9/1
  Curve3/1 -> Display7/1, Multiport Switch/4
  Multiport Switch/1 -> Product3/2, Display1/1

== system Braking_System_2021b/Emetteur/Variant Subsystem/Maitre_Cylindre ==
  Fe_daN : Inport
  Add : Sum  Inputs=+-
  Constant : Constant  Value=pi
  Constant1 : Constant  Value=2
  Constant2 : Constant  Value=100
  Constant3 : Constant
  Constant4 : Constant
  Dia_masterCyl : Constant  Value=maitre_cyl_calcData{5}
  Eff_Ressort : Constant  Value=maitre_cyl_calcData{4}
  Product : Product  Inputs=*/
  Product1 : Product  Inputs=**/
  Product2 : Product  Inputs=*/
  Square : Math  Operator=square  SaturateOnIntegerOverflow=on
  Pe_Bar : Outport
  MC_S_cm² : Outport  Port=2
  Fe_min_daN : Outport  Port=3
  Fe_max_daN : Outport  Port=4
  wires:
  Product2/1 -> Pe_Bar/1
  Constant4/1 -> Fe_max_daN/1
  Constant1/1 -> Product/2
  Constant/1 -> Product1/1
  Square/1 -> Product1/2
  Product/1 -> Square/1
  Constant2/1 -> Product1/3
  Add/1 -> Product2/1
  Eff_Ressort/1 -> Add/2
  Constant3/1 -> Fe_min_daN/1
  Dia_masterCyl/1 -> Product/1
  Product1/1 -> MC_S_cm²/1, Product2/2
  Fe_daN/1 -> Add/1

== system Braking_System_2021b/Emetteur/Variant Subsystem/Valve_HP ==
  note: check out the calculation for the second vavle hp ( no a2, b2 and c2)
  Fe_daN : Inport
  Constant : Constant
  Curve1 : Polyval  Coefs=[valve_hp_calcData{7}, valve_hp_calcData{8}, valve_hp_calcData{9} ]
  Curve2 : Polyval  Coefs=[valve_hp_calcData{11}, valve_hp_calcData{12}, valve_hp_calcData{13} ]
  Curve3 : Polyval  Coefs=[valve_hp_calcData{15}, valve_hp_calcData{16}, valve_hp_calcData{17} ]
  Display{1..3,5..8} (7 alike) : Display
  Gain : Gain  Gain=10
  Multiport Switch : MultiPortSwitch
  Product : Product
  Rendement_ValveHP : Constant  Value=valve_hp_calcData{6}
  valve_k_ch : Subsystem
  Pe_Bar : Outport
  MC_S_cm² : Outport  Port=2
  Fe_min_daN : Outport  Port=3
  Fe_max_daN : Outport  Port=4
  wires:
  Curve1/1 -> Multiport Switch/2, Display5/1
  Multiport Switch/1 -> Display1/1, Product/2
  Fe_daN/1 -> Gain/1
  Product/1 -> Pe_Bar/1, Display2/1
  Rendement_ValveHP/1 -> Product/1
  valve_k_ch/1(Out1) -> Display3/1, Multiport Switch/1
  Constant/1 -> MC_S_cm²/1
  Curve2/1 -> Multiport Switch/3, Display6/1
  Gain/1 -> Curve3/1, valve_k_ch/1(Fe_N), Curve1/1, Curve2/1, Display8/1  "Fe_N"
  Curve3/1 -> Multiport Switch/4, Display7/1

== system Braking_System_2021b/Emetteur/Variant Subsystem/Booster/Booster_k_ch ==
  Fe_N : Inport
  Add1 : Sum  Inputs=+++
  Gain1 : Gain  Gain=3
  Gain2 : Gain  Gain=2
  Product2 : Product
  Relational Operator : RelationalOperator  Operator=<  OutDataTypeStr=boolean  RndMeth=Simplest
  Relational Operator1 : RelationalOperator  Operator=<  OutDataTypeStr=boolean  RndMeth=Simplest
  Relational Operator2 : RelationalOperator  Operator=>  OutDataTypeStr=boolean  RndMeth=Simplest
  Relational Operator3 : RelationalOperator  Operator=>  OutDataTypeStr=boolean  RndMeth=Simplest
  k1 : Constant  Value=booster_k1
  k2 : Constant  Value=booster_k2
  Out1 : Outport
  wires:
  Fe_N/1 -> Relational Operator3/1, Relational Operator1/1, Relational Operator2/1, Relational Operator/1
  Product2/1 -> Gain2/1
  k2/1 -> Relational Operator1/2, Relational Operator3/2
  Relational Operator3/1 -> Gain1/1
  k1/1 -> Relational Operator/2, Relational Operator2/2
  Gain2/1 -> Add1/2
  Relational Operator/1 -> Add1/1
  Gain1/1 -> Add1/3
  Relational Operator2/1 -> Product2/1
  Add1/1 -> Out1/1
  Relational Operator1/1 -> Product2/2

== system Braking_System_2021b/Emetteur/Variant Subsystem/Valve_HP/valve_k_ch ==
  Fe_N : Inport
  Add1 : Sum  Inputs=+++
  Gain1 : Gain  Gain=3
  Gain2 : Gain  Gain=2
  Product2 : Product
  Relational Operator : RelationalOperator  Operator=<  OutDataTypeStr=boolean  RndMeth=Simplest
  Relational Operator1 : RelationalOperator  Operator=<  OutDataTypeStr=boolean  RndMeth=Simplest
  Relational Operator2 : RelationalOperator  Operator=>  OutDataTypeStr=boolean  RndMeth=Simplest
  Relational Operator3 : RelationalOperator  Operator=>  OutDataTypeStr=boolean  RndMeth=Simplest
  k1 : Constant  Value=valve_hp_k1
  k2 : Constant  Value=valve_hp_k2
  Out1 : Outport
  wires:
  Fe_N/1 -> Relational Operator3/1, Relational Operator1/1, Relational Operator2/1, Relational Operator/1
  Product2/1 -> Gain2/1
  k2/1 -> Relational Operator1/2, Relational Operator3/2
  Relational Operator3/1 -> Gain1/1
  k1/1 -> Relational Operator/2, Relational Operator2/2
  Gain2/1 -> Add1/2
  Relational Operator/1 -> Add1/1
  Gain1/1 -> Add1/3
  Relational Operator2/1 -> Product2/1
  Add1/1 -> Out1/1
  Relational Operator1/1 -> Product2/2

== matlab function Braking_System_2021b/Calcul_Laden/MATLAB Function ==
  data: minDecc input; MR output; MR_Min_Dec input; maxBrkDist input; MR_Min_Dist input; Tract input; unbrk_M_Decc input; Target output
function [MR, Target] = fcn(minDecc, MR_Min_Dec, maxBrkDist, MR_Min_Dist, Tract, unbrk_M_Decc)

if minDecc >  MR_Min_Dec && maxBrkDist < MR_Min_Dist && Tract == 1 %strcmp(Tract,"Adhérence")

    MR = 1; %"MR Respected";

else 

    MR = 0; %"MR NOT Respected";

end  



if minDecc >=  unbrk_M_Decc && maxBrkDist <= MR_Min_Dist && Tract == 1 %strcmp(Tract,"Adhérence")

   Target = 1; %"Target Respected";

else 

    Target = 0; %"Target NOT Respected";

end

== matlab function Braking_System_2021b/Calcul_Unladen/MATLAB Function1 ==
  data: minDecc input; MR output; MR_Min_Dec input; maxBrkDist input; MR_Min_Dist input; Tract input; unbrk_M_Decc input; Target output
function [MR, Target] = fcn(minDecc, MR_Min_Dec, maxBrkDist, MR_Min_Dist, Tract, unbrk_M_Decc)

if minDecc >  MR_Min_Dec && maxBrkDist < MR_Min_Dist && Tract == 1 %strcmp(Tract,"Adhérence")

    MR = 1; %"MR Respected";

else 

    MR = 0; %"MR NOT Respected";

end  



if minDecc >=  unbrk_M_Decc && maxBrkDist <= MR_Min_Dist && Tract == 1 %strcmp(Tract,"Adhérence")

   Target = 1; %"Target Respected";

else 

    Target = 0; %"Target NOT Respected";

end
